simulink model "HVDCThyristorBased"  (R2024a)
settings: Solver=FixedStepDiscrete  StartTime=0  StopTime=3  FixedStep=Ts  RelTol=1e-3  AbsTol=1e-2
InitFcn:
  | Ts=50e-6;
  | 
  | % Rectifier AC side :
  | VLL_nom_R = 500e3; % V
  | Fnom_R = 60;           % Hz
  | 
  | % Inverter AC side :
  | VLL_nom_I = 345e3; % V
  | Fnom_I = 50;           % Hz
  | 
  | % DC :
  | Vdc_nom = 500e3;   % V
  | Idc_nom  = 2000;     % A
undefined symbols (not defined in the file or in its folder): D1, Delta, lagging, pulse, test_alpha
libraries: simulink x24, spsOnDelayLib x12, spsFirstOrderFilterLib x9, spsSampleandHoldLib x8, spsBreakerLib x7, spsMultimeterLib x7, spsMonostableLib x7, spsThreePhaseHarmonicFilterLib x6, spsGroundLib x6, spsEdgeDetectorLib x6, spsUniversalBridgeLib x4, spsImpedanceMeasurementLib x3
(part 4 of 5)

== system HVDCThyristorBased/Inverter Control and Protection/Gamma Measurement/Gamma Measurement (Y bridge)/Pulse_counter_sampler (1-6) ==
  angles(1-6) : Inport
  Trigger : TriggerPort  VariantControl=Variant
  Add : Sum
  Constant : Constant  Value=6
  Constant1 : Constant
  Demux : Demux  Outputs=6
  Fcn : Fcn  Expr=(u[1]+1)
  Math Function : Math  Operator=mod  SignedPower=on
  Multiport Switch : MultiPortSwitch  Inputs=6  SaturateOnIntegerOverflow=off  InputSameDT=off
  Unit Delay : UnitDelay  SampleTime=-1  HasFrameUpgradeWarning=on
  angle : Outport  VectorParamsAs1DForOutWhenUnconnected=off
  pulse_n : Outport  Port=2  VectorParamsAs1DForOutWhenUnconnected=off
  wires:
  Demux/6 -> Multiport Switch/7
  Demux/5 -> Multiport Switch/6
  Demux/4 -> Multiport Switch/5
  Demux/3 -> Multiport Switch/4
  Demux/2 -> Multiport Switch/3
  Demux/1 -> Multiport Switch/2
  Fcn/1 -> Unit Delay/1, Math Function/1
  Unit Delay/1 -> Fcn/1
  Constant/1 -> Math Function/2
  Math Function/1 -> Add/2
  Constant1/1 -> Add/1
  Add/1 -> pulse_n/1, Multiport Switch/1
  Multiport Switch/1 -> angle/1
  angles(1-6)/1 -> Demux/1

== system HVDCThyristorBased/Inverter Control and Protection/Gamma Measurement/Gamma Measurement (Y bridge)/Zero crossing interpolation ==
  note: Crossing time error evaluation (t_err) by linear interpolation
      | in a discrete system (sampling time is Ts)
  note: yb
  y : Inport
  Sample : Inport  Port=2
  Enable (Held) : EnablePort  PropagateVarSize=During execution
  (TOL) : simulink/Logic and Bit Operations/Compare To Constant  relop=>=  const=TOL  OutDataTypeStr=boolean  ZeroCross=off
  Abs : Abs
  Constant1 : Constant  Value=y0
  Constant4 : Constant  Value=inf
  Divide : Product  Inputs=*/
  Gain : Gain  Gain=Ts  SaturateOnIntegerOverflow=on  OutDataTypeStr=Inherit: Same as input  ParamDataTypeStr=Inherit: Same as input
  Min+0 Max=Ts : Saturate  UpperLimit=Ts  LowerLimit=0  SampleTime=Ts
  Sample and Hold : spsSampleandHoldLib/Sample and Hold  ic=0  Ts=Ts
  Subtract1 : Sum  Inputs=-+
  Subtract3 : Sum  Inputs=+-
  Switch : Switch  Criteria=u2 > Threshold  OutDataTypeStr=single  SampleTime=Ts
  Unit Delay : UnitDelay  SampleTime=Ts  HasFrameUpgradeWarning=on
  t_err : Outport  VectorParamsAs1DForOutWhenUnconnected=off
  wires:
  Gain/1 -> Divide/1
  Unit Delay/1 -> Subtract3/2  "ya"
  Subtract3/1 -> Abs/1, Switch/1
  Abs/1 -> (TOL)/1
  (TOL)/1 -> Switch/2
  Constant4/1 -> Switch/3
  Switch/1 -> Divide/2
  y/1 -> Unit Delay/1, Subtract3/1, Subtract1/2
  Divide/1 -> Min+0 Max=Ts/1  "correction"
  Constant1/1 -> Subtract1/1
  Subtract1/1 -> Gain/1
  Min+0 Max=Ts/1 -> Sample and Hold/1
  Sample and Hold/1 -> t_err/1
  Sample/1 -> Sample and Hold/2

== system HVDCThyristorBased/Inverter Control and Protection/Inverter Pole Control (Current//Voltage//Gamma)/Current Regulator/PI Regulator with external limits and linrarized Kp (Discrete) ==
  note: PI Regulator With external limits (Linearized Kp) (Discrete)
  Max_i : Inport
  Min_i : Inport  Port=2
  ERR : Inport  Port=3
  Max_pi : Inport  Port=4
  Min_pi : Inport  Port=5
  Alpha_lin : Inport  Port=6
  Max_lin : Inport  Port=7
  Min_lin : Inport  Port=8
  Inv : Inport  Port=9
  Ground : Ground
  Ground1 : Ground
  KI (deg per pu per s) : Gain  Gain=Ki  SaturateOnIntegerOverflow=on  OutDataTypeStr=Inherit: Same as input  ParamDataTypeStr=Inherit: Same as input
  Kp (deg per pu) : Constant  Value=Kp
  Kp Linearisation : Subsystem
  Prod : Product  InputSameDT=on  SaturateOnIntegerOverflow=on  OutDataTypeStr=Inherit: Same as first input
  S16 : Subsystem  mask(Integrator  With  External  Dynamic  Limits (Discrete)){k=1, ic=IC_i, st=pas}
      mask prompts: k "Gain:"; ic "Initial Condition:"; st "Sample time: (s)"
      mask Display: disp('Integrator\nwith\nExternal Limits\nGain & Reset & Hold\n(Discrete)')
  Saturation Dynamic : simulink/Discontinuities/Saturation Dynamic  OutMin=[]  OutMax=[]  OutDataTypeStr=Inherit: Same as second input  OutDataType=fixdt(1, 16)  OutScaling=2^-10  DoSatur=off
  Sum : Sum  InputSameDT=on  SaturateOnIntegerOverflow=on  OutDataTypeStr=Inherit: Same as first input
  Alpha_ord : Outport  InitialOutput=0  VectorParamsAs1DForOutWhenUnconnected=off
  wires:
  Saturation Dynamic/1 -> Alpha_ord/1
  Prod/1 -> Sum/1
  Min_lin/1 -> Kp Linearisation/4(Min_lin)
  Max_lin/1 -> Kp Linearisation/5(Max_lin)
  Inv/1 -> Kp Linearisation/3(Inv)
  ERR/1 -> Prod/2, KI (deg per pu per s)/1
  S16/1(Out) -> Sum/2
  Min_pi/1 -> Saturation Dynamic/3
  Max_pi/1 -> Saturation Dynamic/1
  Sum/1 -> Saturation Dynamic/2
  Min_i/1 -> S16/2(Min)
  Max_i/1 -> S16/1(Max)
  KI (deg per pu per s)/1 -> S16/3(In)
  Kp (deg per pu)/1 -> Kp Linearisation/2(Kp)
  Kp Linearisation/1(Kp_lin) -> Prod/1
  Alpha_lin/1 -> Kp Linearisation/1(Alpha_lin)
  Ground/1 -> S16/4(Reset), S16/5(Hold)
  Ground1/1 -> S16/6(Reset Value)

== system HVDCThyristorBased/Inverter Control and Protection/Inverter Pole Control (Current//Voltage//Gamma)/Gamma Regulator/PI Regulator with external limits and linrarized Kp (Discrete)1 ==
  note: PI Regulator With external limits (Linearized Kp) (Discrete)
  Max_i : Inport
  Min_i : Inport  Port=2
  ERR : Inport  Port=3
  Max_pi : Inport  Port=4
  Min_pi : Inport  Port=5
  Alpha_lin : Inport  Port=6
  Max_lin : Inport  Port=7
  Min_lin : Inport  Port=8
  Inv : Inport  Port=9
  Ground : Ground
  Ground1 : Ground
  KI (deg per pu per s) : Gain  Gain=Ki  SaturateOnIntegerOverflow=on  OutDataTypeStr=Inherit: Same as input  ParamDataTypeStr=Inherit: Same as input
  Kp (deg per pu) : Constant  Value=Kp
  Kp Linearisation : Subsystem
  Prod : Product  InputSameDT=on  SaturateOnIntegerOverflow=on  OutDataTypeStr=Inherit: Same as first input
  S16 : Subsystem  mask(Integrator  With  External  Dynamic  Limits (Discrete)){k=1, ic=IC_i, st=pas}
      mask prompts: k "Gain:"; ic "Initial Condition:"; st "Sample time: (s)"
      mask Display: disp('Integrator\nwith\nExternal Limits\nGain & Reset & Hold\n(Discrete)')
  Saturation Dynamic : simulink/Discontinuities/Saturation Dynamic  OutMin=[]  OutMax=[]  OutDataTypeStr=Inherit: Same as second input  OutDataType=fixdt(1, 16)  OutScaling=2^-10  DoSatur=off
  Sum : Sum  InputSameDT=on  SaturateOnIntegerOverflow=on  OutDataTypeStr=Inherit: Same as first input
  Alpha_ord : Outport  InitialOutput=0  VectorParamsAs1DForOutWhenUnconnected=off
  wires:
  Saturation Dynamic/1 -> Alpha_ord/1
  Prod/1 -> Sum/1
  Min_lin/1 -> Kp Linearisation/4(Min_lin)
  Max_lin/1 -> Kp Linearisation/5(Max_lin)
  Inv/1 -> Kp Linearisation/3(Inv)
  ERR/1 -> Prod/2, KI (deg per pu per s)/1
  S16/1(Out) -> Sum/2
  Min_pi/1 -> Saturation Dynamic/3
  Max_pi/1 -> Saturation Dynamic/1
  Sum/1 -> Saturation Dynamic/2
  Min_i/1 -> S16/2(Min)
  Max_i/1 -> S16/1(Max)
  KI (deg per pu per s)/1 -> S16/3(In)
  Kp (deg per pu)/1 -> Kp Linearisation/2(Kp)
  Kp Linearisation/1(Kp_lin) -> Prod/1
  Alpha_lin/1 -> Kp Linearisation/1(Alpha_lin)
  Ground/1 -> S16/4(Reset), S16/5(Hold)
  Ground1/1 -> S16/6(Reset Value)

== system HVDCThyristorBased/Inverter Control and Protection/Inverter Pole Control (Current//Voltage//Gamma)/Voltage Regulator/PI Regulator with external limits and linrarized Kp (Discrete) ==
  note: PI Regulator With external limits (Linearized Kp) (Discrete)
  Max_i : Inport
  Min_i : Inport  Port=2
  ERR : Inport  Port=3
  Max_pi : Inport  Port=4
  Min_pi : Inport  Port=5
  Alpha_lin : Inport  Port=6
  Max_lin : Inport  Port=7
  Min_lin : Inport  Port=8
  Inv : Inport  Port=9
  Ground : Ground
  Ground1 : Ground
  KI (deg per pu per s) : Gain  Gain=Ki  SaturateOnIntegerOverflow=on  OutDataTypeStr=Inherit: Same as input  ParamDataTypeStr=Inherit: Same as input
  Kp (deg per pu) : Constant  Value=Kp
  Kp Linearisation : Subsystem
  Prod : Product  InputSameDT=on  SaturateOnIntegerOverflow=on  OutDataTypeStr=Inherit: Same as first input
  S16 : Subsystem  mask(Integrator  With  External  Dynamic  Limits (Discrete)){k=1, ic=IC_i, st=pas}
      mask prompts: k "Gain:"; ic "Initial Condition:"; st "Sample time: (s)"
      mask Display: disp('Integrator\nwith\nExternal Limits\nGain & Reset & Hold\n(Discrete)')
  Saturation Dynamic : simulink/Discontinuities/Saturation Dynamic  OutMin=[]  OutMax=[]  OutDataTypeStr=Inherit: Same as second input  OutDataType=fixdt(1, 16)  OutScaling=2^-10  DoSatur=off
  Sum : Sum  InputSameDT=on  SaturateOnIntegerOverflow=on  OutDataTypeStr=Inherit: Same as first input
  Alpha_ord : Outport  InitialOutput=0  VectorParamsAs1DForOutWhenUnconnected=off
  wires:
  Saturation Dynamic/1 -> Alpha_ord/1
  Prod/1 -> Sum/1
  Min_lin/1 -> Kp Linearisation/4(Min_lin)
  Max_lin/1 -> Kp Linearisation/5(Max_lin)
  Inv/1 -> Kp Linearisation/3(Inv)
  ERR/1 -> Prod/2, KI (deg per pu per s)/1
  S16/1(Out) -> Sum/2
  Min_pi/1 -> Saturation Dynamic/3
  Max_pi/1 -> Saturation Dynamic/1
  Sum/1 -> Saturation Dynamic/2
  Min_i/1 -> S16/2(Min)
  Max_i/1 -> S16/1(Max)
  KI (deg per pu per s)/1 -> S16/3(In)
  Kp (deg per pu)/1 -> Kp Linearisation/2(Kp)
  Kp Linearisation/1(Kp_lin) -> Prod/1
  Alpha_lin/1 -> Kp Linearisation/1(Alpha_lin)
  Ground/1 -> S16/4(Reset), S16/5(Hold)
  Ground1/1 -> S16/6(Reset Value)

== system HVDCThyristorBased/Inverter Control and Protection/Inverter Pole Control (Current//Voltage//Gamma)/Voltage dependent Current Order Limiter/Low Pass (IC = 1.0) ==
  note: Low Pass Filter
      | with external Tc & Reset
      | (Zoh methode)
  note: Silvano Casoria
      | Power System Simulation Laboratory
      |  IREQ, Hydro-Quebec
  In : Inport
  R : Inport  Port=2
  T : Inport  Port=3
  Constant : Constant  Value=Ts
  IC= ic : UnitDelay  InitialCondition=ic  SampleTime=dt  HasFrameUpgradeWarning=on
  Math Function : Math  Operator=reciprocal  SignedPower=on
  Product : Product  Inputs=3  InputSameDT=on  SaturateOnIntegerOverflow=on  OutDataTypeStr=Inherit: Same as first input
  Sum : Sum  Inputs=+-  InputSameDT=on  SaturateOnIntegerOverflow=on  OutDataTypeStr=Inherit: Same as first input
  Sum1 : Sum  InputSameDT=on  SaturateOnIntegerOverflow=on  OutDataTypeStr=Inherit: Same as first input
  Switch : Switch  Criteria=u2 > Threshold
  Out : Outport  VectorParamsAs1DForOutWhenUnconnected=off
  wires:
  IC= ic/1 -> Sum/2, Sum1/2
  In/1 -> Switch/1, Sum/1
  Sum1/1 -> Out/1, Switch/3
  Switch/1 -> IC= ic/1
  Product/1 -> Sum1/1
  Sum/1 -> Product/2
  Math Function/1 -> Product/1
  T/1 -> Math Function/1
  Constant/1 -> Product/3
  R/1 -> Switch/2

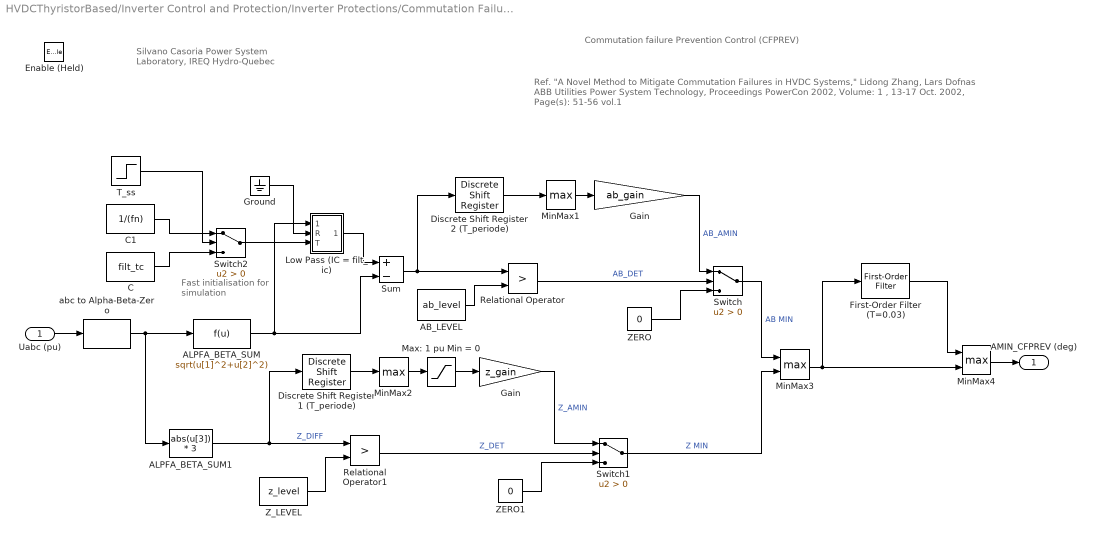
== system HVDCThyristorBased/Inverter Control and Protection/Inverter Protections/Commutation Failure Prevention Control (CFPREV)/CFPREV ==
  note: Ref. "A Novel Method to Mitigate Commutation Failures in HVDC Systems,"
      | Lidong Zhang, Lars Dofnas ABB Utilities Power System Technology,
      | Proceedings PowerCon 2002, Volume: 1 , 13-17 Oct. 2002,  Page(s): 51-56 vol.1
  note: Silvano Casoria
      | Power System Laboratory, IREQ
      | Hydro-Quebec
  note: Commutation failure Prevention Control (CFPREV)
  note: Fast initialisation
      | for simulation
  Uabc (pu) : Inport
  Enable (Held) : EnablePort  PropagateVarSize=During execution
  AB_LEVEL : Constant  Value=ab_level
  ALPFA_BETA_SUM : Fcn  Expr=sqrt(u[1]^2+u[2]^2)
  ALPFA_BETA_SUM1 : Fcn  Expr=abs(u[3]) * 3
  C : Constant  Value=filt_tc
  C1 : Constant  Value=1/(fn)
  Discrete Shift Register 1 (T_periode) : spsDiscreteShiftRegisterLib/Discrete Shift Register  NSamples=fix(T_periode/Ts)  InitialValue=0  Ts=Ts
  Discrete Shift Register 2 (T_periode) : spsDiscreteShiftRegisterLib/Discrete Shift Register  NSamples=fix(T_periode/Ts)  InitialValue=0  Ts=Ts
  First-Order Filter (T=0.03) : spsFirstOrderFilterLib/First-Order Filter  FilterType=Lowpass  Tc=0.03  Ts=Ts  Initialize=off  Vac_Init=[0, 0, Fnom_I]  Vdc_Init=0  PlotResponse=off  FreqRange="[0,  200,  1]"
  Gain : Gain  Gain=ab_gain  SaturateOnIntegerOverflow=on  OutDataTypeStr=Inherit: Same as input  ParamDataTypeStr=Inherit: Same as input
  "Gain  " : Gain  Gain=z_gain  SaturateOnIntegerOverflow=on  OutDataTypeStr=Inherit: Same as input  ParamDataTypeStr=Inherit: Same as input
  Ground : Ground
  Low Pass (IC = filt_ic) : Subsystem  mask(Low Pass Filter With Reset (discrete: Zoh method, Forward Euler)){ic=filt_ic, dt=Ts}
      mask prompts: ic "Initial condition:"; dt "Sample time (s)"
      mask help:
      | The output will be reset to the input value (Time constant = 0)  during the input (2) is True. The Time constant (T) is defined by
      | input (3).
      mask Display:
      | plot(0,0,100,100,[90,80,70,60,50,40,29,20,10],[60,55,52,55,60,65,67,65,60],[89,80,71,60,50,40,30,20,10],[40,35,32,35,40,45,47,45,40],[56,44],[70,50]);
      | disp('\n\nD')
  Max: 1 pu Min = 0 : Saturate  UpperLimit=1.0  LowerLimit=0
  MinMax1 : MinMax  Function=max  InputSameDT=on  SaturateOnIntegerOverflow=on
  MinMax2 : MinMax  Function=max  InputSameDT=on  SaturateOnIntegerOverflow=on
  MinMax3 : MinMax  Function=max  Inputs=2  InputSameDT=on  SaturateOnIntegerOverflow=on
  MinMax4 : MinMax  Function=max  Inputs=2  InputSameDT=on  SaturateOnIntegerOverflow=on
  Relational Operator : RelationalOperator  Operator=>  InputSameDT=off
  Relational Operator1 : RelationalOperator  Operator=>  InputSameDT=off
  Sum : Sum  Inputs=+-  SaturateOnIntegerOverflow=on
  Switch : Switch  Criteria=u2 > Threshold  InputSameDT=off
  Switch1 : Switch  Criteria=u2 > Threshold  InputSameDT=off
  Switch2 : Switch  Criteria=u2 > Threshold  InputSameDT=off
  T_ss : Step  Time=T_ss  Before=1  After=0  SampleTime=0
  ZERO : Constant  Value=0
  ZERO1 : Constant  Value=0
  Z_LEVEL : Constant  Value=z_level
  abc to Alpha-Beta-Zero : spsabctoAlphaBetaZeroLib/abc to Alpha-Beta-Zero
  AMIN_CFPREV (deg) : Outport  VectorParamsAs1DForOutWhenUnconnected=off
  wires:
  MinMax4/1 -> AMIN_CFPREV (deg)/1
  MinMax3/1 -> First-Order Filter (T=0.03)/1, MinMax4/2
  ALPFA_BETA_SUM/1 -> Low Pass (IC = filt_ic)/1(In), Sum/2
  Sum/1 -> Discrete Shift Register 2 (T_periode)/1, Relational Operator/1
  AB_LEVEL/1 -> Relational Operator/2
  Relational Operator/1 -> Switch/2  "AB_DET"
  Discrete Shift Register 2 (T_periode)/1 -> MinMax1/1
  MinMax1/1 -> Gain/1
  Gain/1 -> Switch/1  "AB_AMIN"
  ZERO/1 -> Switch/3
  ALPFA_BETA_SUM1/1 -> Discrete Shift Register 1 (T_periode)/1, Relational Operator1/1  "Z_DIFF"
  Z_LEVEL/1 -> Relational Operator1/2
  Discrete Shift Register 1 (T_periode)/1 -> MinMax2/1
  MinMax2/1 -> Max: 1 pu Min = 0/1
  Max: 1 pu Min = 0/1 -> "Gain  "/1
  Relational Operator1/1 -> Switch1/2  "Z_DET"
  "Gain  "/1 -> Switch1/1  "Z_AMIN"
  ZERO1/1 -> Switch1/3
  Switch/1 -> MinMax3/1  "AB MIN"
  Switch1/1 -> MinMax3/2  "Z MIN"
  abc to Alpha-Beta-Zero/1 -> ALPFA_BETA_SUM/1, ALPFA_BETA_SUM1/1
  Uabc (pu)/1 -> abc to Alpha-Beta-Zero/1
  Low Pass (IC = filt_ic)/1(Out) -> Sum/1
  Switch2/1 -> Low Pass (IC = filt_ic)/3(T)
  C/1 -> Switch2/3
  T_ss/1 -> Switch2/2
  C1/1 -> Switch2/1
  Ground/1 -> Low Pass (IC = filt_ic)/2(R)
  First-Order Filter (T=0.03)/1 -> MinMax4/1

== system HVDCThyristorBased/Inverter Control and Protection/Inverter Protections/Low  AC Voltage Detection (LACVD)/LACVD ==
  note: Low AC Voltage Detection
  Uac (pu) : Inport
  Enable (Held) : EnablePort  PropagateVarSize=During execution
  Off Delay : spsOnDelayLib/On Delay  DelayType=Off delay  delay=0.009  ic=0  Ts=Ts
  "On Delay 1 " : spsOnDelayLib/On Delay  DelayType=On delay  delay=0.001  ic=0  Ts=Ts
  On Delay 2 : spsOnDelayLib/On Delay  DelayType=On delay  delay=0.014  ic=0  Ts=Ts
  REF_1 (pu) : Constant  Value=Ref_1
  Relational Operator1 : RelationalOperator  Operator=<=
  Low_AC_Voltage : Outport  VectorParamsAs1DForOutWhenUnconnected=off
  wires:
  REF_1 (pu)/1 -> Relational Operator1/2
  Uac (pu)/1 -> Relational Operator1/1
  "On Delay 1 "/1 -> Off Delay/1
  Off Delay/1 -> On Delay 2/1
  Relational Operator1/1 -> "On Delay 1 "/1
  On Delay 2/1 -> Low_AC_Voltage/1

== system HVDCThyristorBased/Rectifier Control and Protection/Rectifier Pole Control (Current)/Current Regulator/PI Regulator with external limits and linrarized Kp (Discrete) ==
  note: PI Regulator With external limits (Linearized Kp) (Discrete)
  Max_i : Inport
  Min_i : Inport  Port=2
  ERR : Inport  Port=3
  Max_pi : Inport  Port=4
  Min_pi : Inport  Port=5
  Alpha_lin : Inport  Port=6
  Max_lin : Inport  Port=7
  Min_lin : Inport  Port=8
  Inv : Inport  Port=9
  Ground : Ground
  Ground1 : Ground
  KI (deg per pu per s) : Gain  Gain=Ki  SaturateOnIntegerOverflow=on  OutDataTypeStr=Inherit: Same as input  ParamDataTypeStr=Inherit: Same as input
  Kp (deg per pu) : Constant  Value=Kp
  Kp Linearisation : Subsystem
  Prod : Product  InputSameDT=on  SaturateOnIntegerOverflow=on  OutDataTypeStr=Inherit: Same as first input
  S16 : Subsystem  mask(Integrator  With  External  Dynamic  Limits (Discrete)){k=1, ic=IC_i, st=pas}
      mask prompts: k "Gain:"; ic "Initial Condition:"; st "Sample time: (s)"
      mask Display: disp('Integrator\nwith\nExternal Limits\nGain & Reset & Hold\n(Discrete)')
  Saturation Dynamic : simulink/Discontinuities/Saturation Dynamic  OutMin=[]  OutMax=[]  OutDataTypeStr=Inherit: Same as second input  OutDataType=fixdt(1, 16)  OutScaling=2^-10  DoSatur=off
  Sum : Sum  InputSameDT=on  SaturateOnIntegerOverflow=on  OutDataTypeStr=Inherit: Same as first input
  Alpha_ord : Outport  InitialOutput=0  VectorParamsAs1DForOutWhenUnconnected=off
  wires:
  Saturation Dynamic/1 -> Alpha_ord/1
  Prod/1 -> Sum/1
  Min_lin/1 -> Kp Linearisation/4(Min_lin)
  Max_lin/1 -> Kp Linearisation/5(Max_lin)
  Inv/1 -> Kp Linearisation/3(Inv)
  ERR/1 -> Prod/2, KI (deg per pu per s)/1
  S16/1(Out) -> Sum/2
  Min_pi/1 -> Saturation Dynamic/3
  Max_pi/1 -> Saturation Dynamic/1
  Sum/1 -> Saturation Dynamic/2
  Min_i/1 -> S16/2(Min)
  Max_i/1 -> S16/1(Max)
  KI (deg per pu per s)/1 -> S16/3(In)
  Kp (deg per pu)/1 -> Kp Linearisation/2(Kp)
  Kp Linearisation/1(Kp_lin) -> Prod/1
  Alpha_lin/1 -> Kp Linearisation/1(Alpha_lin)
  Ground/1 -> S16/4(Reset), S16/5(Hold)
  Ground1/1 -> S16/6(Reset Value)

== system HVDCThyristorBased/Rectifier Control and Protection/Rectifier Pole Control (Current)/Gamma Regulator/PI Regulator with external limits and linrarized Kp (Discrete)1 ==
  note: PI Regulator With external limits (Linearized Kp) (Discrete)
  Max_i : Inport
  Min_i : Inport  Port=2
  ERR : Inport  Port=3
  Max_pi : Inport  Port=4
  Min_pi : Inport  Port=5
  Alpha_lin : Inport  Port=6
  Max_lin : Inport  Port=7
  Min_lin : Inport  Port=8
  Inv : Inport  Port=9
  Ground : Ground
  Ground1 : Ground
  KI (deg per pu per s) : Gain  Gain=Ki  SaturateOnIntegerOverflow=on  OutDataTypeStr=Inherit: Same as input  ParamDataTypeStr=Inherit: Same as input
  Kp (deg per pu) : Constant  Value=Kp
  Kp Linearisation : Subsystem
  Prod : Product  InputSameDT=on  SaturateOnIntegerOverflow=on  OutDataTypeStr=Inherit: Same as first input
  S16 : Subsystem  mask(Integrator  With  External  Dynamic  Limits (Discrete)){k=1, ic=IC_i, st=pas}
      mask prompts: k "Gain:"; ic "Initial Condition:"; st "Sample time: (s)"
      mask Display: disp('Integrator\nwith\nExternal Limits\nGain & Reset & Hold\n(Discrete)')
  Saturation Dynamic : simulink/Discontinuities/Saturation Dynamic  OutMin=[]  OutMax=[]  OutDataTypeStr=Inherit: Same as second input  OutDataType=fixdt(1, 16)  OutScaling=2^-10  DoSatur=off
  Sum : Sum  InputSameDT=on  SaturateOnIntegerOverflow=on  OutDataTypeStr=Inherit: Same as first input
  Alpha_ord : Outport  InitialOutput=0  VectorParamsAs1DForOutWhenUnconnected=off
  wires:
  Saturation Dynamic/1 -> Alpha_ord/1
  Prod/1 -> Sum/1
  Min_lin/1 -> Kp Linearisation/4(Min_lin)
  Max_lin/1 -> Kp Linearisation/5(Max_lin)
  Inv/1 -> Kp Linearisation/3(Inv)
  ERR/1 -> Prod/2, KI (deg per pu per s)/1
  S16/1(Out) -> Sum/2
  Min_pi/1 -> Saturation Dynamic/3
  Max_pi/1 -> Saturation Dynamic/1
  Sum/1 -> Saturation Dynamic/2
  Min_i/1 -> S16/2(Min)
  Max_i/1 -> S16/1(Max)
  KI (deg per pu per s)/1 -> S16/3(In)
  Kp (deg per pu)/1 -> Kp Linearisation/2(Kp)
  Kp Linearisation/1(Kp_lin) -> Prod/1
  Alpha_lin/1 -> Kp Linearisation/1(Alpha_lin)
  Ground/1 -> S16/4(Reset), S16/5(Hold)
  Ground1/1 -> S16/6(Reset Value)

== system HVDCThyristorBased/Rectifier Control and Protection/Rectifier Pole Control (Current)/Voltage Regulator/PI Regulator with external limits and linrarized Kp (Discrete) ==
  note: PI Regulator With external limits (Linearized Kp) (Discrete)
  Max_i : Inport
  Min_i : Inport  Port=2
  ERR : Inport  Port=3
  Max_pi : Inport  Port=4
  Min_pi : Inport  Port=5
  Alpha_lin : Inport  Port=6
  Max_lin : Inport  Port=7
  Min_lin : Inport  Port=8
  Inv : Inport  Port=9
  Ground : Ground
  Ground1 : Ground
  KI (deg per pu per s) : Gain  Gain=Ki  SaturateOnIntegerOverflow=on  OutDataTypeStr=Inherit: Same as input  ParamDataTypeStr=Inherit: Same as input
  Kp (deg per pu) : Constant  Value=Kp
  Kp Linearisation : Subsystem
  Prod : Product  InputSameDT=on  SaturateOnIntegerOverflow=on  OutDataTypeStr=Inherit: Same as first input
  S16 : Subsystem  mask(Integrator  With  External  Dynamic  Limits (Discrete)){k=1, ic=IC_i, st=pas}
      mask prompts: k "Gain:"; ic "Initial Condition:"; st "Sample time: (s)"
      mask Display: disp('Integrator\nwith\nExternal Limits\nGain & Reset & Hold\n(Discrete)')
  Saturation Dynamic : simulink/Discontinuities/Saturation Dynamic  OutMin=[]  OutMax=[]  OutDataTypeStr=Inherit: Same as second input  OutDataType=fixdt(1, 16)  OutScaling=2^-10  DoSatur=off
  Sum : Sum  InputSameDT=on  SaturateOnIntegerOverflow=on  OutDataTypeStr=Inherit: Same as first input
  Alpha_ord : Outport  InitialOutput=0  VectorParamsAs1DForOutWhenUnconnected=off
  wires:
  Saturation Dynamic/1 -> Alpha_ord/1
  Prod/1 -> Sum/1
  Min_lin/1 -> Kp Linearisation/4(Min_lin)
  Max_lin/1 -> Kp Linearisation/5(Max_lin)
  Inv/1 -> Kp Linearisation/3(Inv)
  ERR/1 -> Prod/2, KI (deg per pu per s)/1
  S16/1(Out) -> Sum/2
  Min_pi/1 -> Saturation Dynamic/3
  Max_pi/1 -> Saturation Dynamic/1
  Sum/1 -> Saturation Dynamic/2
  Min_i/1 -> S16/2(Min)
  Max_i/1 -> S16/1(Max)
  KI (deg per pu per s)/1 -> S16/3(In)
  Kp (deg per pu)/1 -> Kp Linearisation/2(Kp)
  Kp Linearisation/1(Kp_lin) -> Prod/1
  Alpha_lin/1 -> Kp Linearisation/1(Alpha_lin)
  Ground/1 -> S16/4(Reset), S16/5(Hold)
  Ground1/1 -> S16/6(Reset Value)

== system HVDCThyristorBased/Rectifier Control and Protection/Rectifier Pole Control (Current)/Voltage dependent Current Order Limiter/Low Pass (IC = 1.0) ==
  note: Low Pass Filter
      | with external Tc & Reset
      | (Zoh methode)
  note: Silvano Casoria
      | Power System Simulation Laboratory
      |  IREQ, Hydro-Quebec
  In : Inport
  R : Inport  Port=2
  T : Inport  Port=3
  Constant : Constant  Value=Ts
  IC= ic : UnitDelay  InitialCondition=ic  SampleTime=dt  HasFrameUpgradeWarning=on
  Math Function : Math  Operator=reciprocal  SignedPower=on
  Product : Product  Inputs=3  InputSameDT=on  SaturateOnIntegerOverflow=on  OutDataTypeStr=Inherit: Same as first input
  Sum : Sum  Inputs=+-  InputSameDT=on  SaturateOnIntegerOverflow=on  OutDataTypeStr=Inherit: Same as first input
  Sum1 : Sum  InputSameDT=on  SaturateOnIntegerOverflow=on  OutDataTypeStr=Inherit: Same as first input
  Switch : Switch  Criteria=u2 > Threshold
  Out : Outport  VectorParamsAs1DForOutWhenUnconnected=off
  wires:
  IC= ic/1 -> Sum/2, Sum1/2
  In/1 -> Switch/1, Sum/1
  Sum1/1 -> Out/1, Switch/3
  Switch/1 -> IC= ic/1
  Product/1 -> Sum1/1
  Sum/1 -> Product/2
  Math Function/1 -> Product/1
  T/1 -> Math Function/1
  Constant/1 -> Product/3
  R/1 -> Switch/2

== system HVDCThyristorBased/Rectifier Control and Protection/Rectifier Protections/DC Fault Protection (DCPROT)/Enabled Subsystem ==
  note: DC Fault Protection (only in Rectifier)
  VdL (pu) : Inport
  Deblocked : Inport  Port=2  OutDataTypeStr=boolean
  Lock : Inport  Port=3
  Enable (Held) : EnablePort  PropagateVarSize=During execution
  Data Type Conversion : DataTypeConversion  OutDataTypeStr=boolean
  Logical Operator2 : Logic  Inputs=3
  Logical Operator3 : Logic  Operator=NOT
  Logical Operator6 : Logic
  Monostable (T=T2) : spsMonostableLib/Monostable  EdgeDetect=Rising  PulseDuration=T2  ic=0  Ts=Ts
  ON: -Ref1 (pu) OFF: -(Ref1+0.1) : Relay  OnSwitchValue=-Ref1  OffSwitchValue=-(Ref1 + 0.1)
  "Off Delay 1 " : spsOnDelayLib/On Delay  DelayType=Off delay  delay=0.01  ic=0  Ts=Ts
  Off Delay 2 : spsOnDelayLib/On Delay  DelayType=Off delay  delay=0.16  ic=0  Ts=Ts
  On Delay : spsOnDelayLib/On Delay  DelayType=On delay  delay=0.2  ic=0  Ts=Ts
  On Delay (T=T1) : spsOnDelayLib/On Delay  DelayType=On delay  delay=T1  ic=0  Ts=Ts
  minus : Gain  Gain=-1  SaturateOnIntegerOverflow=on  OutDataTypeStr=Inherit: Same as input  ParamDataTypeStr=Inherit: Same as input
  voltage sign (pole +) : Gain  Gain=sign  SaturateOnIntegerOverflow=on  OutDataTypeStr=Inherit: Same as input  ParamDataTypeStr=Inherit: Same as input
  Forced_alpha : Outport  VectorParamsAs1DForOutWhenUnconnected=off
  wires:
  minus/1 -> ON: -Ref1 (pu) OFF: -(Ref1+0.1)/1
  Data Type Conversion/1 -> Logical Operator6/1
  On Delay/1 -> Logical Operator6/2
  Logical Operator6/1 -> "Off Delay 1 "/1
  ON: -Ref1 (pu) OFF: -(Ref1+0.1)/1 -> Data Type Conversion/1
  Deblocked/1 -> On Delay/1, Logical Operator2/3
  VdL (pu)/1 -> voltage sign (pole +)/1  "VdL"
  voltage sign (pole +)/1 -> minus/1
  Logical Operator3/1 -> Logical Operator2/2
  Logical Operator2/1 -> On Delay (T=T1)/1
  On Delay (T=T1)/1 -> Monostable (T=T2)/1
  Monostable (T=T2)/1 -> Forced_alpha/1
  "Off Delay 1 "/1 -> Logical Operator2/1
  Lock/1 -> Off Delay 2/1
  Off Delay 2/1 -> Logical Operator3/1

== system HVDCThyristorBased/Rectifier Control and Protection/Rectifier Protections/Low  AC Voltage Detection (LACVD)/LACVD ==
  note: Low AC Voltage Detection
  Uac (pu) : Inport
  Enable (Held) : EnablePort  PropagateVarSize=During execution
  Off Delay : spsOnDelayLib/On Delay  DelayType=Off delay  delay=0.009  ic=0  Ts=Ts
  "On Delay 1 " : spsOnDelayLib/On Delay  DelayType=On delay  delay=0.001  ic=0  Ts=Ts
  On Delay 2 : spsOnDelayLib/On Delay  DelayType=On delay  delay=0.014  ic=0  Ts=Ts
  REF_1 (pu) : Constant  Value=Ref_1
  Relational Operator1 : RelationalOperator  Operator=<=
  Low_AC_Voltage : Outport  VectorParamsAs1DForOutWhenUnconnected=off
  wires:
  REF_1 (pu)/1 -> Relational Operator1/2
  Uac (pu)/1 -> Relational Operator1/1
  "On Delay 1 "/1 -> Off Delay/1
  Off Delay/1 -> On Delay 2/1
  Relational Operator1/1 -> "On Delay 1 "/1
  On Delay 2/1 -> Low_AC_Voltage/1

== system HVDCThyristorBased/Inverter Control and Protection/Inverter Pole Control (Current//Voltage//Gamma)/Current Regulator/PI Regulator with external limits and linrarized Kp (Discrete)/Kp Linearisation ==
  note: Kp Linearization
  Alpha_lin : Inport
  Kp : Inport  Port=2
  Inv : Inport  Port=3
  Min_lin : Inport  Port=4
  Max_lin : Inport  Port=5
  Constant3 : Constant  Value=On_lin
  Data Type Conversion : DataTypeConversion  OutDataTypeStr=boolean
  Logical Operator : Logic  Operator=NOT
  Logical Operator1 : Logic  Operator=NOT
  Math Function : Math  Operator=reciprocal  SignedPower=on
  Prod2 : Product  Inputs=3  InputSameDT=on  SaturateOnIntegerOverflow=on  OutDataTypeStr=Inherit: Same as first input
  Saturation Dynamic : simulink/Discontinuities/Saturation Dynamic  OutMin=[]  OutMax=[]  OutDataTypeStr=Inherit: Same as second input  OutDataType=fixdt(1, 16)  OutScaling=2^-10  DoSatur=off
  Switch : Switch  Criteria=u2 > Threshold
  Switch1 : Switch  Criteria=u2 > Threshold
  Trigonometric Function : Trigonometry
  Trigonometric Function1 : Trigonometry
  k : Gain  Gain=pi/180  SaturateOnIntegerOverflow=on  OutDataTypeStr=Inherit: Same as input  ParamDataTypeStr=Inherit: Same as input
  k1 : Gain  Gain=pi/180  SaturateOnIntegerOverflow=on  OutDataTypeStr=Inherit: Same as input  ParamDataTypeStr=Inherit: Same as input
  Kp_lin : Outport  InitialOutput=0  VectorParamsAs1DForOutWhenUnconnected=off
  wires:
  Min_lin/1 -> Switch/1, Saturation Dynamic/3
  Max_lin/1 -> Saturation Dynamic/1, Switch/3
  Alpha_lin/1 -> Saturation Dynamic/2
  Math Function/1 -> Prod2/2
  Trigonometric Function1/1 -> Math Function/1
  k/1 -> Trigonometric Function1/1
  Kp/1 -> Switch1/1, Prod2/3
  Inv/1 -> Logical Operator/1
  Logical Operator/1 -> Switch/2
  Trigonometric Function/1 -> Prod2/1
  Saturation Dynamic/1 -> k/1
  k1/1 -> Trigonometric Function/1
  Switch/1 -> k1/1
  Switch1/1 -> Kp_lin/1
  Prod2/1 -> Switch1/3
  Logical Operator1/1 -> Switch1/2  "off"
  Constant3/1 -> Data Type Conversion/1
  Data Type Conversion/1 -> Logical Operator1/1

== system HVDCThyristorBased/Inverter Control and Protection/Inverter Pole Control (Current//Voltage//Gamma)/Current Regulator/PI Regulator with external limits and linrarized Kp (Discrete)/S16 ==
  note: INTEGRATOR with External limits & Reset & Hold
  note: Gain * Ts
  Max : Inport
  Min : Inport  Port=2
  In : Inport  Port=3
  Reset : Inport  Port=4
  Hold : Inport  Port=5
  Reset Value : Inport  Port=6
  Gain1 : Gain  Gain=k*st  SaturateOnIntegerOverflow=on  OutDataTypeStr=Inherit: Same as input  ParamDataTypeStr=Inherit: Same as input
  IC = ic : UnitDelay  InitialCondition=ic  SampleTime=st  HasFrameUpgradeWarning=on
  Logical Operator4 : Logic  Operator=OR
  MinMax : MinMax  Inputs=2  InputSameDT=on  SaturateOnIntegerOverflow=on
  MinMax1 : MinMax  Function=max  Inputs=2  InputSameDT=on  SaturateOnIntegerOverflow=on
  Saturation Dynamic : simulink/Discontinuities/Saturation Dynamic  OutMin=[]  OutMax=[]  OutDataTypeStr=Inherit: Same as second input  OutDataType=fixdt(1, 16)  OutScaling=2^-10  DoSatur=off
  Sum : Sum  InputSameDT=on  SaturateOnIntegerOverflow=on  OutDataTypeStr=Inherit: Same as first input
  Switch2 : Switch  Criteria=u2 > Threshold
  Switch3 : Switch  Criteria=u2 > Threshold
  Switch7 : Switch  Criteria=u2 > Threshold
  Out : Outport  InitialOutput=0  VectorParamsAs1DForOutWhenUnconnected=off
  wires:
  Saturation Dynamic/1 -> Out/1, IC = ic/1
  Gain1/1 -> Sum/1
  In/1 -> Gain1/1
  Sum/1 -> Saturation Dynamic/2
  Hold/1 -> Logical Operator4/1
  Reset/1 -> Switch7/2, Logical Operator4/2
  Logical Operator4/1 -> Switch2/2, Switch3/2
  Switch2/1 -> MinMax/1
  Max/1 -> Switch2/3, MinMax/2
  Reset Value/1 -> Switch7/1
  MinMax/1 -> Saturation Dynamic/1
  MinMax1/1 -> Saturation Dynamic/3
  Switch3/1 -> MinMax1/1
  Min/1 -> Switch3/3, MinMax1/2
  IC = ic/1 -> Switch7/3
  Switch7/1 -> Switch3/1, Sum/2, Switch2/1

== system HVDCThyristorBased/Inverter Control and Protection/Inverter Pole Control (Current//Voltage//Gamma)/Gamma Regulator/PI Regulator with external limits and linrarized Kp (Discrete)1/Kp Linearisation ==
  note: Kp Linearization
  Alpha_lin : Inport
  Kp : Inport  Port=2
  Inv : Inport  Port=3
  Min_lin : Inport  Port=4
  Max_lin : Inport  Port=5
  Constant3 : Constant  Value=On_lin
  Data Type Conversion : DataTypeConversion  OutDataTypeStr=boolean
  Logical Operator : Logic  Operator=NOT
  Logical Operator1 : Logic  Operator=NOT
  Math Function : Math  Operator=reciprocal  SignedPower=on
  Prod2 : Product  Inputs=3  InputSameDT=on  SaturateOnIntegerOverflow=on  OutDataTypeStr=Inherit: Same as first input
  Saturation Dynamic : simulink/Discontinuities/Saturation Dynamic  OutMin=[]  OutMax=[]  OutDataTypeStr=Inherit: Same as second input  OutDataType=fixdt(1, 16)  OutScaling=2^-10  DoSatur=off
  Switch : Switch  Criteria=u2 > Threshold
  Switch1 : Switch  Criteria=u2 > Threshold
  Trigonometric Function : Trigonometry
  Trigonometric Function1 : Trigonometry
  k : Gain  Gain=pi/180  SaturateOnIntegerOverflow=on  OutDataTypeStr=Inherit: Same as input  ParamDataTypeStr=Inherit: Same as input
  k1 : Gain  Gain=pi/180  SaturateOnIntegerOverflow=on  OutDataTypeStr=Inherit: Same as input  ParamDataTypeStr=Inherit: Same as input
  Kp_lin : Outport  InitialOutput=0  VectorParamsAs1DForOutWhenUnconnected=off
  wires:
  Min_lin/1 -> Switch/1, Saturation Dynamic/3
  Max_lin/1 -> Saturation Dynamic/1, Switch/3
  Alpha_lin/1 -> Saturation Dynamic/2
  Math Function/1 -> Prod2/2
  Trigonometric Function1/1 -> Math Function/1
  k/1 -> Trigonometric Function1/1
  Kp/1 -> Switch1/1, Prod2/3
  Inv/1 -> Logical Operator/1
  Logical Operator/1 -> Switch/2
  Trigonometric Function/1 -> Prod2/1
  Saturation Dynamic/1 -> k/1
  k1/1 -> Trigonometric Function/1
  Switch/1 -> k1/1
  Switch1/1 -> Kp_lin/1
  Prod2/1 -> Switch1/3
  Logical Operator1/1 -> Switch1/2  "off"
  Constant3/1 -> Data Type Conversion/1
  Data Type Conversion/1 -> Logical Operator1/1

== system HVDCThyristorBased/Inverter Control and Protection/Inverter Pole Control (Current//Voltage//Gamma)/Gamma Regulator/PI Regulator with external limits and linrarized Kp (Discrete)1/S16 ==
  note: INTEGRATOR with External limits & Reset & Hold
  note: Gain * Ts
  Max : Inport
  Min : Inport  Port=2
  In : Inport  Port=3
  Reset : Inport  Port=4
  Hold : Inport  Port=5
  Reset Value : Inport  Port=6
  Gain1 : Gain  Gain=k*st  SaturateOnIntegerOverflow=on  OutDataTypeStr=Inherit: Same as input  ParamDataTypeStr=Inherit: Same as input
  IC = ic : UnitDelay  InitialCondition=ic  SampleTime=st  HasFrameUpgradeWarning=on
  Logical Operator4 : Logic  Operator=OR
  MinMax : MinMax  Inputs=2  InputSameDT=on  SaturateOnIntegerOverflow=on
  MinMax1 : MinMax  Function=max  Inputs=2  InputSameDT=on  SaturateOnIntegerOverflow=on
  Saturation Dynamic : simulink/Discontinuities/Saturation Dynamic  OutMin=[]  OutMax=[]  OutDataTypeStr=Inherit: Same as second input  OutDataType=fixdt(1, 16)  OutScaling=2^-10  DoSatur=off
  Sum : Sum  InputSameDT=on  SaturateOnIntegerOverflow=on  OutDataTypeStr=Inherit: Same as first input
  Switch2 : Switch  Criteria=u2 > Threshold
  Switch3 : Switch  Criteria=u2 > Threshold
  Switch7 : Switch  Criteria=u2 > Threshold
  Out : Outport  InitialOutput=0  VectorParamsAs1DForOutWhenUnconnected=off
  wires:
  Saturation Dynamic/1 -> Out/1, IC = ic/1
  Gain1/1 -> Sum/1
  In/1 -> Gain1/1
  Sum/1 -> Saturation Dynamic/2
  Hold/1 -> Logical Operator4/1
  Reset/1 -> Switch7/2, Logical Operator4/2
  Logical Operator4/1 -> Switch2/2, Switch3/2
  Switch2/1 -> MinMax/1
  Max/1 -> Switch2/3, MinMax/2
  Reset Value/1 -> Switch7/1
  MinMax/1 -> Saturation Dynamic/1
  MinMax1/1 -> Saturation Dynamic/3
  Switch3/1 -> MinMax1/1
  Min/1 -> Switch3/3, MinMax1/2
  IC = ic/1 -> Switch7/3
  Switch7/1 -> Switch3/1, Sum/2, Switch2/1

== system HVDCThyristorBased/Inverter Control and Protection/Inverter Pole Control (Current//Voltage//Gamma)/Voltage Regulator/PI Regulator with external limits and linrarized Kp (Discrete)/Kp Linearisation ==
  note: Kp Linearization
  Alpha_lin : Inport
  Kp : Inport  Port=2
  Inv : Inport  Port=3
  Min_lin : Inport  Port=4
  Max_lin : Inport  Port=5
  Constant3 : Constant  Value=On_lin
  Data Type Conversion : DataTypeConversion  OutDataTypeStr=boolean
  Logical Operator : Logic  Operator=NOT
  Logical Operator1 : Logic  Operator=NOT
  Math Function : Math  Operator=reciprocal  SignedPower=on
  Prod2 : Product  Inputs=3  InputSameDT=on  SaturateOnIntegerOverflow=on  OutDataTypeStr=Inherit: Same as first input
  Saturation Dynamic : simulink/Discontinuities/Saturation Dynamic  OutMin=[]  OutMax=[]  OutDataTypeStr=Inherit: Same as second input  OutDataType=fixdt(1, 16)  OutScaling=2^-10  DoSatur=off
  Switch : Switch  Criteria=u2 > Threshold
  Switch1 : Switch  Criteria=u2 > Threshold
  Trigonometric Function : Trigonometry
  Trigonometric Function1 : Trigonometry
  k : Gain  Gain=pi/180  SaturateOnIntegerOverflow=on  OutDataTypeStr=Inherit: Same as input  ParamDataTypeStr=Inherit: Same as input
  k1 : Gain  Gain=pi/180  SaturateOnIntegerOverflow=on  OutDataTypeStr=Inherit: Same as input  ParamDataTypeStr=Inherit: Same as input
  Kp_lin : Outport  InitialOutput=0  VectorParamsAs1DForOutWhenUnconnected=off
  wires:
  Min_lin/1 -> Switch/1, Saturation Dynamic/3
  Max_lin/1 -> Saturation Dynamic/1, Switch/3
  Alpha_lin/1 -> Saturation Dynamic/2
  Math Function/1 -> Prod2/2
  Trigonometric Function1/1 -> Math Function/1
  k/1 -> Trigonometric Function1/1
  Kp/1 -> Switch1/1, Prod2/3
  Inv/1 -> Logical Operator/1
  Logical Operator/1 -> Switch/2
  Trigonometric Function/1 -> Prod2/1
  Saturation Dynamic/1 -> k/1
  k1/1 -> Trigonometric Function/1
  Switch/1 -> k1/1
  Switch1/1 -> Kp_lin/1
  Prod2/1 -> Switch1/3
  Logical Operator1/1 -> Switch1/2  "off"
  Constant3/1 -> Data Type Conversion/1
  Data Type Conversion/1 -> Logical Operator1/1

== system HVDCThyristorBased/Inverter Control and Protection/Inverter Pole Control (Current//Voltage//Gamma)/Voltage Regulator/PI Regulator with external limits and linrarized Kp (Discrete)/S16 ==
  note: INTEGRATOR with External limits & Reset & Hold
  note: Gain * Ts
  Max : Inport
  Min : Inport  Port=2
  In : Inport  Port=3
  Reset : Inport  Port=4
  Hold : Inport  Port=5
  Reset Value : Inport  Port=6
  Gain1 : Gain  Gain=k*st  SaturateOnIntegerOverflow=on  OutDataTypeStr=Inherit: Same as input  ParamDataTypeStr=Inherit: Same as input
  IC = ic : UnitDelay  InitialCondition=ic  SampleTime=st  HasFrameUpgradeWarning=on
  Logical Operator4 : Logic  Operator=OR
  MinMax : MinMax  Inputs=2  InputSameDT=on  SaturateOnIntegerOverflow=on
  MinMax1 : MinMax  Function=max  Inputs=2  InputSameDT=on  SaturateOnIntegerOverflow=on
  Saturation Dynamic : simulink/Discontinuities/Saturation Dynamic  OutMin=[]  OutMax=[]  OutDataTypeStr=Inherit: Same as second input  OutDataType=fixdt(1, 16)  OutScaling=2^-10  DoSatur=off
  Sum : Sum  InputSameDT=on  SaturateOnIntegerOverflow=on  OutDataTypeStr=Inherit: Same as first input
  Switch2 : Switch  Criteria=u2 > Threshold
  Switch3 : Switch  Criteria=u2 > Threshold
  Switch7 : Switch  Criteria=u2 > Threshold
  Out : Outport  InitialOutput=0  VectorParamsAs1DForOutWhenUnconnected=off
  wires:
  Saturation Dynamic/1 -> Out/1, IC = ic/1
  Gain1/1 -> Sum/1
  In/1 -> Gain1/1
  Sum/1 -> Saturation Dynamic/2
  Hold/1 -> Logical Operator4/1
  Reset/1 -> Switch7/2, Logical Operator4/2
  Logical Operator4/1 -> Switch2/2, Switch3/2
  Switch2/1 -> MinMax/1
  Max/1 -> Switch2/3, MinMax/2
  Reset Value/1 -> Switch7/1
  MinMax/1 -> Saturation Dynamic/1
  MinMax1/1 -> Saturation Dynamic/3
  Switch3/1 -> MinMax1/1
  Min/1 -> Switch3/3, MinMax1/2
  IC = ic/1 -> Switch7/3
  Switch7/1 -> Switch3/1, Sum/2, Switch2/1

== system HVDCThyristorBased/Inverter Control and Protection/Inverter Protections/Commutation Failure Prevention Control (CFPREV)/CFPREV/Low Pass (IC = filt_ic) ==
  note: Low Pass Filter
      | with external Tc & Reset
      | (Zoh methode)
  note: Silvano Casoria
      | Power System Simulation Laboratory
      |  IREQ, Hydro-Quebec
  In : Inport
  R : Inport  Port=2
  T : Inport  Port=3
  Constant : Constant  Value=Ts
  IC= ic : UnitDelay  InitialCondition=ic  SampleTime=dt  HasFrameUpgradeWarning=on
  Math Function : Math  Operator=reciprocal  SignedPower=on
  Product : Product  Inputs=3  InputSameDT=on  SaturateOnIntegerOverflow=on  OutDataTypeStr=Inherit: Same as first input
  Sum : Sum  Inputs=+-  InputSameDT=on  SaturateOnIntegerOverflow=on  OutDataTypeStr=Inherit: Same as first input
  Sum1 : Sum  InputSameDT=on  SaturateOnIntegerOverflow=on  OutDataTypeStr=Inherit: Same as first input
  Switch : Switch  Criteria=u2 > Threshold
  Out : Outport  VectorParamsAs1DForOutWhenUnconnected=off
  wires:
  IC= ic/1 -> Sum/2, Sum1/2
  In/1 -> Switch/1, Sum/1
  Sum1/1 -> Out/1, Switch/3
  Switch/1 -> IC= ic/1
  Product/1 -> Sum1/1
  Sum/1 -> Product/2
  Math Function/1 -> Product/1
  T/1 -> Math Function/1
  Constant/1 -> Product/3
  R/1 -> Switch/2

== system HVDCThyristorBased/Rectifier Control and Protection/Rectifier Pole Control (Current)/Current Regulator/PI Regulator with external limits and linrarized Kp (Discrete)/Kp Linearisation ==
  note: Kp Linearization
  Alpha_lin : Inport
  Kp : Inport  Port=2
  Inv : Inport  Port=3
  Min_lin : Inport  Port=4
  Max_lin : Inport  Port=5
  Constant3 : Constant  Value=On_lin
  Data Type Conversion : DataTypeConversion  OutDataTypeStr=boolean
  Logical Operator : Logic  Operator=NOT
  Logical Operator1 : Logic  Operator=NOT
  Math Function : Math  Operator=reciprocal  SignedPower=on
  Prod2 : Product  Inputs=3  InputSameDT=on  SaturateOnIntegerOverflow=on  OutDataTypeStr=Inherit: Same as first input
  Saturation Dynamic : simulink/Discontinuities/Saturation Dynamic  OutMin=[]  OutMax=[]  OutDataTypeStr=Inherit: Same as second input  OutDataType=fixdt(1, 16)  OutScaling=2^-10  DoSatur=off
  Switch : Switch  Criteria=u2 > Threshold
  Switch1 : Switch  Criteria=u2 > Threshold
  Trigonometric Function : Trigonometry
  Trigonometric Function1 : Trigonometry
  k : Gain  Gain=pi/180  SaturateOnIntegerOverflow=on  OutDataTypeStr=Inherit: Same as input  ParamDataTypeStr=Inherit: Same as input
  k1 : Gain  Gain=pi/180  SaturateOnIntegerOverflow=on  OutDataTypeStr=Inherit: Same as input  ParamDataTypeStr=Inherit: Same as input
  Kp_lin : Outport  InitialOutput=0  VectorParamsAs1DForOutWhenUnconnected=off
  wires:
  Min_lin/1 -> Switch/1, Saturation Dynamic/3
  Max_lin/1 -> Saturation Dynamic/1, Switch/3
  Alpha_lin/1 -> Saturation Dynamic/2
  Math Function/1 -> Prod2/2
  Trigonometric Function1/1 -> Math Function/1
  k/1 -> Trigonometric Function1/1
  Kp/1 -> Switch1/1, Prod2/3
  Inv/1 -> Logical Operator/1
  Logical Operator/1 -> Switch/2
  Trigonometric Function/1 -> Prod2/1
  Saturation Dynamic/1 -> k/1
  k1/1 -> Trigonometric Function/1
  Switch/1 -> k1/1
  Switch1/1 -> Kp_lin/1
  Prod2/1 -> Switch1/3
  Logical Operator1/1 -> Switch1/2  "off"
  Constant3/1 -> Data Type Conversion/1
  Data Type Conversion/1 -> Logical Operator1/1

== system HVDCThyristorBased/Rectifier Control and Protection/Rectifier Pole Control (Current)/Current Regulator/PI Regulator with external limits and linrarized Kp (Discrete)/S16 ==
  note: INTEGRATOR with External limits & Reset & Hold
  note: Gain * Ts
  Max : Inport
  Min : Inport  Port=2
  In : Inport  Port=3
  Reset : Inport  Port=4
  Hold : Inport  Port=5
  Reset Value : Inport  Port=6
  Gain1 : Gain  Gain=k*st  SaturateOnIntegerOverflow=on  OutDataTypeStr=Inherit: Same as input  ParamDataTypeStr=Inherit: Same as input
  IC = ic : UnitDelay  InitialCondition=ic  SampleTime=st  HasFrameUpgradeWarning=on
  Logical Operator4 : Logic  Operator=OR
  MinMax : MinMax  Inputs=2  InputSameDT=on  SaturateOnIntegerOverflow=on
  MinMax1 : MinMax  Function=max  Inputs=2  InputSameDT=on  SaturateOnIntegerOverflow=on
  Saturation Dynamic : simulink/Discontinuities/Saturation Dynamic  OutMin=[]  OutMax=[]  OutDataTypeStr=Inherit: Same as second input  OutDataType=fixdt(1, 16)  OutScaling=2^-10  DoSatur=off
  Sum : Sum  InputSameDT=on  SaturateOnIntegerOverflow=on  OutDataTypeStr=Inherit: Same as first input
  Switch2 : Switch  Criteria=u2 > Threshold
  Switch3 : Switch  Criteria=u2 > Threshold
  Switch7 : Switch  Criteria=u2 > Threshold
  Out : Outport  InitialOutput=0  VectorParamsAs1DForOutWhenUnconnected=off
  wires:
  Saturation Dynamic/1 -> Out/1, IC = ic/1
  Gain1/1 -> Sum/1
  In/1 -> Gain1/1
  Sum/1 -> Saturation Dynamic/2
  Hold/1 -> Logical Operator4/1
  Reset/1 -> Switch7/2, Logical Operator4/2
  Logical Operator4/1 -> Switch2/2, Switch3/2
  Switch2/1 -> MinMax/1
  Max/1 -> Switch2/3, MinMax/2
  Reset Value/1 -> Switch7/1
  MinMax/1 -> Saturation Dynamic/1
  MinMax1/1 -> Saturation Dynamic/3
  Switch3/1 -> MinMax1/1
  Min/1 -> Switch3/3, MinMax1/2
  IC = ic/1 -> Switch7/3
  Switch7/1 -> Switch3/1, Sum/2, Switch2/1

== system HVDCThyristorBased/Rectifier Control and Protection/Rectifier Pole Control (Current)/Gamma Regulator/PI Regulator with external limits and linrarized Kp (Discrete)1/Kp Linearisation ==
  note: Kp Linearization
  Alpha_lin : Inport
  Kp : Inport  Port=2
  Inv : Inport  Port=3
  Min_lin : Inport  Port=4
  Max_lin : Inport  Port=5
  Constant3 : Constant  Value=On_lin
  Data Type Conversion : DataTypeConversion  OutDataTypeStr=boolean
  Logical Operator : Logic  Operator=NOT
  Logical Operator1 : Logic  Operator=NOT
  Math Function : Math  Operator=reciprocal  SignedPower=on
  Prod2 : Product  Inputs=3  InputSameDT=on  SaturateOnIntegerOverflow=on  OutDataTypeStr=Inherit: Same as first input
  Saturation Dynamic : simulink/Discontinuities/Saturation Dynamic  OutMin=[]  OutMax=[]  OutDataTypeStr=Inherit: Same as second input  OutDataType=fixdt(1, 16)  OutScaling=2^-10  DoSatur=off
  Switch : Switch  Criteria=u2 > Threshold
  Switch1 : Switch  Criteria=u2 > Threshold
  Trigonometric Function : Trigonometry
  Trigonometric Function1 : Trigonometry
  k : Gain  Gain=pi/180  SaturateOnIntegerOverflow=on  OutDataTypeStr=Inherit: Same as input  ParamDataTypeStr=Inherit: Same as input
  k1 : Gain  Gain=pi/180  SaturateOnIntegerOverflow=on  OutDataTypeStr=Inherit: Same as input  ParamDataTypeStr=Inherit: Same as input
  Kp_lin : Outport  InitialOutput=0  VectorParamsAs1DForOutWhenUnconnected=off
  wires:
  Min_lin/1 -> Switch/1, Saturation Dynamic/3
  Max_lin/1 -> Saturation Dynamic/1, Switch/3
  Alpha_lin/1 -> Saturation Dynamic/2
  Math Function/1 -> Prod2/2
  Trigonometric Function1/1 -> Math Function/1
  k/1 -> Trigonometric Function1/1
  Kp/1 -> Switch1/1, Prod2/3
  Inv/1 -> Logical Operator/1
  Logical Operator/1 -> Switch/2
  Trigonometric Function/1 -> Prod2/1
  Saturation Dynamic/1 -> k/1
  k1/1 -> Trigonometric Function/1
  Switch/1 -> k1/1
  Switch1/1 -> Kp_lin/1
  Prod2/1 -> Switch1/3
  Logical Operator1/1 -> Switch1/2  "off"
  Constant3/1 -> Data Type Conversion/1
  Data Type Conversion/1 -> Logical Operator1/1

== system HVDCThyristorBased/Rectifier Control and Protection/Rectifier Pole Control (Current)/Gamma Regulator/PI Regulator with external limits and linrarized Kp (Discrete)1/S16 ==
  note: INTEGRATOR with External limits & Reset & Hold
  note: Gain * Ts
  Max : Inport
  Min : Inport  Port=2
  In : Inport  Port=3
  Reset : Inport  Port=4
  Hold : Inport  Port=5
  Reset Value : Inport  Port=6
  Gain1 : Gain  Gain=k*st  SaturateOnIntegerOverflow=on  OutDataTypeStr=Inherit: Same as input  ParamDataTypeStr=Inherit: Same as input
  IC = ic : UnitDelay  InitialCondition=ic  SampleTime=st  HasFrameUpgradeWarning=on
  Logical Operator4 : Logic  Operator=OR
  MinMax : MinMax  Inputs=2  InputSameDT=on  SaturateOnIntegerOverflow=on
  MinMax1 : MinMax  Function=max  Inputs=2  InputSameDT=on  SaturateOnIntegerOverflow=on
  Saturation Dynamic : simulink/Discontinuities/Saturation Dynamic  OutMin=[]  OutMax=[]  OutDataTypeStr=Inherit: Same as second input  OutDataType=fixdt(1, 16)  OutScaling=2^-10  DoSatur=off
  Sum : Sum  InputSameDT=on  SaturateOnIntegerOverflow=on  OutDataTypeStr=Inherit: Same as first input
  Switch2 : Switch  Criteria=u2 > Threshold
  Switch3 : Switch  Criteria=u2 > Threshold
  Switch7 : Switch  Criteria=u2 > Threshold
  Out : Outport  InitialOutput=0  VectorParamsAs1DForOutWhenUnconnected=off
  wires:
  Saturation Dynamic/1 -> Out/1, IC = ic/1
  Gain1/1 -> Sum/1
  In/1 -> Gain1/1
  Sum/1 -> Saturation Dynamic/2
  Hold/1 -> Logical Operator4/1
  Reset/1 -> Switch7/2, Logical Operator4/2
  Logical Operator4/1 -> Switch2/2, Switch3/2
  Switch2/1 -> MinMax/1
  Max/1 -> Switch2/3, MinMax/2
  Reset Value/1 -> Switch7/1
  MinMax/1 -> Saturation Dynamic/1
  MinMax1/1 -> Saturation Dynamic/3
  Switch3/1 -> MinMax1/1
  Min/1 -> Switch3/3, MinMax1/2
  IC = ic/1 -> Switch7/3
  Switch7/1 -> Switch3/1, Sum/2, Switch2/1
